simulink model "raspiHostFlightGearVisualization"  (R2021b)
settings: Solver=FixedStepDiscrete  StartTime=0.0  StopTime=inf  RelTol=1e-3  EnableMultiTasking=on
undefined symbols (not defined in the file): f
libraries: FlightGearLib x1, instrumentlib x1
settings Model: Creator=promero  LastModifiedBy=promero
settings SolverCC: ConcurrentTasks=on  AlgebraicLoopSolver=TrustRegion  InsertRTBMode=Never (minimum delay)
settings DebuggingCC: SFMachineParentedDataDiag=warning
settings SFSimCC: CustomCodeUndefinedFunction=UseInterfaceOnly

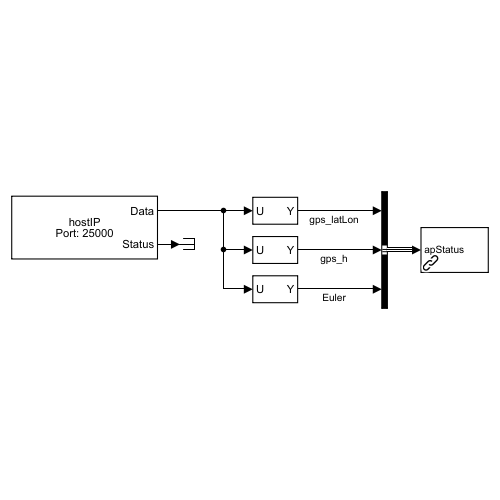
[thumbnail: Simulink's stored preview of the top-level diagram]
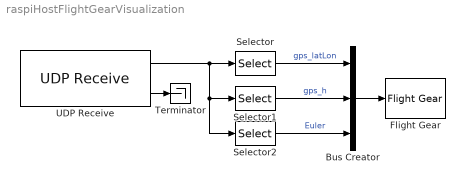
== system raspiHostFlightGearVisualization ==
  Bus Creator : BusCreator  Inputs=3
  Flight Gear : FlightGearLib/Flight Gear  SystemSampleTime=-1  VariantControl=animMode == 2  VariantActivationTime=update diagram  Latency=0  AutoFrameSizeCalculation=off
  Selector : Selector  InputPortWidth=6  IndexOptions=Index vector (dialog)  Indices=[1 2]  OutputSizes=1
  Selector1 : Selector  InputPortWidth=6  IndexOptions=Index vector (dialog)  Indices=3  OutputSizes=1
  Selector2 : Selector  InputPortWidth=6  IndexOptions=Index vector (dialog)  Indices=[4 5 6]  OutputSizes=1
  Terminator : Terminator
  UDP Receive : instrumentlib/UDP Receive  Host=raspiIP  Port=9090  LocalPort=25000  EnablePortSharing=off  GetLatestData=on  DataSize=6  DataType=single  ASCIIFormatting=%f,  Terminator=LF  ByteOrder=BigEndian  EnableBlockingMode=off  Timeout=10  SampleTime=-1  LocalAddress=hostIP
  wires:
  Bus Creator/1 -> Flight Gear/1
  UDP Receive/2 -> Terminator/1
  UDP Receive/1 -> Selector2/1, Selector1/1, Selector/1
  Selector/1 -> Bus Creator/1  "gps_latLon"
  Selector1/1 -> Bus Creator/2  "gps_h"
  Selector2/1 -> Bus Creator/3  "Euler"
